simulink model "testConstantWECMotion"  (R2022a)
settings: Solver=VariableStepAuto  StartTime=0.0  StopTime=10.0  MaxStep=0.001  RelTol=1e-3
settings Model: Creator=simmo536  LastModifiedBy=simmo536

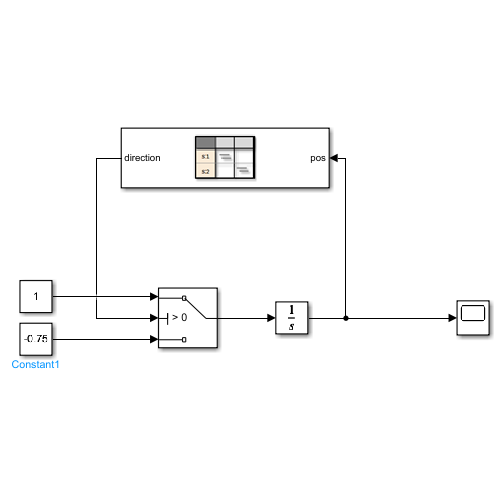
[thumbnail: Simulink's stored preview of the top-level diagram]
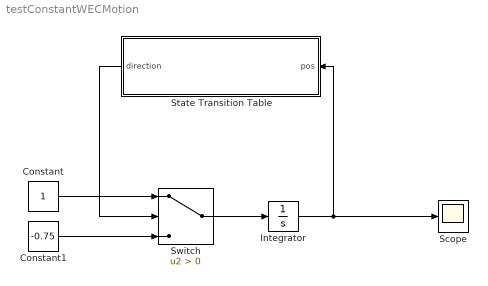
== system testConstantWECMotion ==
  Constant : Constant
  Constant1 : Constant  Value=-0.75
  Integrator : Integrator
  Scope : Scope
  State Transition Table : State Transition Table  TreatAsAtomicUnit=on
  Switch : Switch  Criteria=u2 > Threshold  SaturateOnIntegerOverflow=off  InputSameDT=off
  wires:
  State Transition Table/1(direction) -> Switch/2
  Switch/1 -> Integrator/1
  Integrator/1 -> State Transition Table/1(pos), Scope/1
  Constant/1 -> Switch/1
  Constant1/1 -> Switch/3

== stateflow chart testConstantWECMotion/State Transition Table ==
  state forward
    entry:
    direction=1;
  state reverse
    entry:
    direction=0;
  (default) -> forward
  forward -> (junction 25) [order 2] : [pos<WEC_positiveLimit]
  (junction 25) -> forward
  forward -> reverse [order 1] : [pos>=WEC_positiveLimit]
  reverse -> forward [order 1] : [pos<=WEC_negativeLimit]
  reverse -> (junction 29) [order 2] : [pos>WEC_negativeLimit]
  (junction 29) -> reverse
  data: pos input; direction output; WEC_negativeLimit constant double =-1; WEC_positiveLimit constant double =1
